simulink model "stdp_pattern3x3_training_2023noclock"  (R2024a)
settings: Solver=FixedStepAuto  StartTime=0.0  StopTime=2  FixedStep=0.000005  RelTol=1e-3
model workspace (MAT data in the model file):
  part1_v1 = 1
values from neighbouring files (symbols this model uses):
  full_pattern = load('Pattern4_250.CSV')    [model_setup4.m]
  max_weight2 = 255    [model_setup4.m]
  min_weight2 = 150    [model_setup4.m]
  Th_control_time2 = 0.02    [model_setup4.m]    (also in model_setup_test.m = 2)
  Th_minus_count2 = 10    [model_setup4.m]    (also in model_setup_test.m = 5)
  Th_plus_count2 = 20    [model_setup4.m]    (also in model_setup_test.m)
libraries: simulink x1
(part 3 of 9)

== system stdp_pattern3x3_training_2023noclock/Synapse22 ==
  note: weight 초기값
  note: pre spike trace
  note: weight 최댓값
  note: STDP
  note: Synapse
  note: weight 최솟값
  note: post spike trace
  note: 기존 weight + STDP 변화량
  note: weight RC 감소
  Pre_spike : Inport
  addr : Inport  Port=2
  Post_spike : Inport  Port=3
  Add1 : Sum
  Clock1 : Subsystem
  Clock2 : Subsystem
  Clock3 : Subsystem
  Delay1 : Delay  DelayLength=1  SampleTime=0.00001
  Exp : Math
  Exp1 : Math
  From Workspace : FromWorkspace  VariableName=Rand_var
  From Workspace1 : FromWorkspace  VariableName=min_weight
  From Workspace2 : FromWorkspace  VariableName=max_weight
  From Workspace3 : FromWorkspace  VariableName=synapse_weight_rc_s
  From Workspace4 : FromWorkspace  VariableName=synapse_weight_rc_l
  From Workspace6 : FromWorkspace  VariableName=initial_LTP
  From Workspace7 : FromWorkspace  VariableName=initial_LTD
  From Workspace8 : FromWorkspace  VariableName=RC_LTP
  From Workspace9 : FromWorkspace  VariableName=RC_LTD
  Gain1 : Gain  Gain=-1
  MATLAB Function1 : MATLAB Function  TreatAsAtomicUnit=on
  Memory1 : Memory
  Memory2 : Memory
  OR : Logic  Operator=OR  IconShape=distinctive  AllPortsSameDT=off  OutDataTypeStr=boolean
  Product{,1..6} (7 alike) : Product
  Scope1 : Scope  NumInputPorts=4
  Scope2 : Scope  NumInputPorts=5
  Scope3 : Scope  NumInputPorts=2
  Scope5 : Scope  NumInputPorts=3
  Scope6 : Scope  NumInputPorts=3
  Scope7 : Scope  NumInputPorts=3
  Scope8 : Scope  NumInputPorts=4
  Subsystem : Subsystem
  Switch : Switch  Threshold=max_weight2  SaturateOnIntegerOverflow=off  InputSameDT=off
  Switch1 : Switch  Criteria=u2 > Threshold  Threshold=min_weight2  SaturateOnIntegerOverflow=off  InputSameDT=off
  rc_add1 : MATLAB Function  TreatAsAtomicUnit=on
  rc_add2 : MATLAB Function  TreatAsAtomicUnit=on
  Weight : Outport
  Spike_out : Outport  Port=2
  Weight_out : Outport  Port=3
  wires:
  Switch1/1 -> Scope7/3, Product/2, Weight_out/1, Scope5/3, Scope3/1, Delay1/1
  Product/1 -> Memory1/1
  addr/1 -> MATLAB Function1/2(synapse_num)
  Post_spike/1 -> Scope2/4, Memory2/1
  Clock1/1(T) -> rc_add2/1(tx)
  Clock2/1(T) -> Scope2/3, rc_add1/1(ty)
  Delay1/1 -> Scope3/2, Subsystem/2(before_weight), Scope6/3
  Memory1/1 -> Weight/1, Scope5/2
  From Workspace7/1 -> rc_add1/2(initial_LTD)
  From Workspace9/1 -> rc_add1/3(tau_LTD)
  From Workspace6/1 -> rc_add2/2(initial_LTP)
  From Workspace8/1 -> rc_add2/3(tau_LTP)
  Product6/1 -> Scope1/4, Add1/2
  Product5/1 -> Scope1/2, Add1/1
  Add1/1 -> Subsystem/1(delta_weight), Scope2/1, Scope6/1
  From Workspace2/1 -> Product3/2
  Product2/1 -> Exp1/1
  Gain1/1 -> Product1/2, Product2/1
  From Workspace1/1 -> Switch1/3
  Exp1/1 -> Scope8/2, Product4/2
  Switch/1 -> Scope8/4, Switch1/2, Scope7/2, Switch1/1
  From Workspace3/1 -> Product2/2
  Product3/1 -> Switch/1
  Exp/1 -> Product3/1
  Clock3/1(T) -> Gain1/1
  Product1/1 -> Exp/1
  MATLAB Function1/1(y) -> Scope6/2, Product4/1, Scope7/1, Switch/2, Scope8/1
  From Workspace4/1 -> Product1/1
  From Workspace/1 -> MATLAB Function1/1(init_weight)
  Product4/1 -> Scope8/3, Switch/3
  Subsystem/1(weight) -> MATLAB Function1/3(before_weight)
  rc_add2/1(pre_trace) -> Product5/1, Scope1/1
  rc_add1/1(post_trace) -> Product6/2, Scope1/3
  OR/1 -> Subsystem/Trigger
  Memory2/1 -> OR/2, Product5/2, Clock2/1("Reset "), Scope2/5
  Pre_spike/1 -> OR/1, Scope5/1, Spike_out/1, Product/1, Clock3/1("Reset "), Clock1/1("Reset "), Product6/1, Scope2/2

== system stdp_pattern3x3_training_2023noclock/Synapse23 ==
  note: weight 초기값
  note: pre spike trace
  note: weight 최댓값
  note: STDP
  note: Synapse
  note: weight 최솟값
  note: post spike trace
  note: 기존 weight + STDP 변화량
  note: weight RC 감소
  Pre_spike : Inport
  addr : Inport  Port=2
  Post_spike : Inport  Port=3
  Add1 : Sum
  Clock1 : Subsystem
  Clock2 : Subsystem
  Clock3 : Subsystem
  Delay1 : Delay  DelayLength=1  SampleTime=0.00001
  Exp : Math
  Exp1 : Math
  From Workspace : FromWorkspace  VariableName=Rand_var
  From Workspace1 : FromWorkspace  VariableName=min_weight
  From Workspace2 : FromWorkspace  VariableName=max_weight
  From Workspace3 : FromWorkspace  VariableName=synapse_weight_rc_s
  From Workspace4 : FromWorkspace  VariableName=synapse_weight_rc_l
  From Workspace6 : FromWorkspace  VariableName=initial_LTP
  From Workspace7 : FromWorkspace  VariableName=initial_LTD
  From Workspace8 : FromWorkspace  VariableName=RC_LTP
  From Workspace9 : FromWorkspace  VariableName=RC_LTD
  Gain1 : Gain  Gain=-1
  MATLAB Function1 : MATLAB Function  TreatAsAtomicUnit=on
  Memory1 : Memory
  Memory2 : Memory
  OR : Logic  Operator=OR  IconShape=distinctive  AllPortsSameDT=off  OutDataTypeStr=boolean
  Product{,1..6} (7 alike) : Product
  Scope1 : Scope  NumInputPorts=4
  Scope2 : Scope  NumInputPorts=5
  Scope3 : Scope  NumInputPorts=2
  Scope5 : Scope  NumInputPorts=3
  Scope6 : Scope  NumInputPorts=3
  Scope7 : Scope  NumInputPorts=3
  Scope8 : Scope  NumInputPorts=4
  Subsystem : Subsystem
  Switch : Switch  Threshold=max_weight2  SaturateOnIntegerOverflow=off  InputSameDT=off
  Switch1 : Switch  Criteria=u2 > Threshold  Threshold=min_weight2  SaturateOnIntegerOverflow=off  InputSameDT=off
  rc_add1 : MATLAB Function  TreatAsAtomicUnit=on
  rc_add2 : MATLAB Function  TreatAsAtomicUnit=on
  Weight : Outport
  Spike_out : Outport  Port=2
  Weight_out : Outport  Port=3
  wires:
  Switch1/1 -> Scope7/3, Product/2, Weight_out/1, Scope5/3, Scope3/1, Delay1/1
  Product/1 -> Memory1/1
  addr/1 -> MATLAB Function1/2(synapse_num)
  Post_spike/1 -> Scope2/4, Memory2/1
  Clock1/1(T) -> rc_add2/1(tx)
  Clock2/1(T) -> Scope2/3, rc_add1/1(ty)
  Delay1/1 -> Scope3/2, Subsystem/2(before_weight), Scope6/3
  Memory1/1 -> Weight/1, Scope5/2
  From Workspace7/1 -> rc_add1/2(initial_LTD)
  From Workspace9/1 -> rc_add1/3(tau_LTD)
  From Workspace6/1 -> rc_add2/2(initial_LTP)
  From Workspace8/1 -> rc_add2/3(tau_LTP)
  Product6/1 -> Scope1/4, Add1/2
  Product5/1 -> Scope1/2, Add1/1
  Add1/1 -> Subsystem/1(delta_weight), Scope2/1, Scope6/1
  From Workspace2/1 -> Product3/2
  Product2/1 -> Exp1/1
  Gain1/1 -> Product1/2, Product2/1
  From Workspace1/1 -> Switch1/3
  Exp1/1 -> Scope8/2, Product4/2
  Switch/1 -> Scope8/4, Switch1/2, Scope7/2, Switch1/1
  From Workspace3/1 -> Product2/2
  Product3/1 -> Switch/1
  Exp/1 -> Product3/1
  Clock3/1(T) -> Gain1/1
  Product1/1 -> Exp/1
  MATLAB Function1/1(y) -> Scope6/2, Product4/1, Scope7/1, Switch/2, Scope8/1
  From Workspace4/1 -> Product1/1
  From Workspace/1 -> MATLAB Function1/1(init_weight)
  Product4/1 -> Scope8/3, Switch/3
  Subsystem/1(weight) -> MATLAB Function1/3(before_weight)
  rc_add2/1(pre_trace) -> Product5/1, Scope1/1
  rc_add1/1(post_trace) -> Product6/2, Scope1/3
  OR/1 -> Subsystem/Trigger
  Memory2/1 -> OR/2, Product5/2, Clock2/1("Reset "), Scope2/5
  Pre_spike/1 -> OR/1, Scope5/1, Spike_out/1, Product/1, Clock3/1("Reset "), Clock1/1("Reset "), Product6/1, Scope2/2

== system stdp_pattern3x3_training_2023noclock/Synapse24 ==
  note: weight 초기값
  note: pre spike trace
  note: weight 최댓값
  note: STDP
  note: Synapse
  note: weight 최솟값
  note: post spike trace
  note: 기존 weight + STDP 변화량
  note: weight RC 감소
  Pre_spike : Inport
  addr : Inport  Port=2
  Post_spike : Inport  Port=3
  Add1 : Sum
  Clock1 : Subsystem
  Clock2 : Subsystem
  Clock3 : Subsystem
  Delay1 : Delay  DelayLength=1  SampleTime=0.00001
  Exp : Math
  Exp1 : Math
  From Workspace : FromWorkspace  VariableName=Rand_var
  From Workspace1 : FromWorkspace  VariableName=min_weight
  From Workspace2 : FromWorkspace  VariableName=max_weight
  From Workspace3 : FromWorkspace  VariableName=synapse_weight_rc_s
  From Workspace4 : FromWorkspace  VariableName=synapse_weight_rc_l
  From Workspace6 : FromWorkspace  VariableName=initial_LTP
  From Workspace7 : FromWorkspace  VariableName=initial_LTD
  From Workspace8 : FromWorkspace  VariableName=RC_LTP
  From Workspace9 : FromWorkspace  VariableName=RC_LTD
  Gain1 : Gain  Gain=-1
  MATLAB Function1 : MATLAB Function  TreatAsAtomicUnit=on
  Memory1 : Memory
  Memory2 : Memory
  OR : Logic  Operator=OR  IconShape=distinctive  AllPortsSameDT=off  OutDataTypeStr=boolean
  Product{,1..6} (7 alike) : Product
  Scope1 : Scope  NumInputPorts=4
  Scope2 : Scope  NumInputPorts=5
  Scope3 : Scope  NumInputPorts=2
  Scope5 : Scope  NumInputPorts=3
  Scope6 : Scope  NumInputPorts=3
  Scope7 : Scope  NumInputPorts=3
  Scope8 : Scope  NumInputPorts=4
  Subsystem : Subsystem
  Switch : Switch  Threshold=max_weight2  SaturateOnIntegerOverflow=off  InputSameDT=off
  Switch1 : Switch  Criteria=u2 > Threshold  Threshold=min_weight2  SaturateOnIntegerOverflow=off  InputSameDT=off
  rc_add1 : MATLAB Function  TreatAsAtomicUnit=on
  rc_add2 : MATLAB Function  TreatAsAtomicUnit=on
  Weight : Outport
  Spike_out : Outport  Port=2
  Weight_out : Outport  Port=3
  wires:
  Switch1/1 -> Scope7/3, Product/2, Weight_out/1, Scope5/3, Scope3/1, Delay1/1
  Product/1 -> Memory1/1
  addr/1 -> MATLAB Function1/2(synapse_num)
  Post_spike/1 -> Scope2/4, Memory2/1
  Clock1/1(T) -> rc_add2/1(tx)
  Clock2/1(T) -> Scope2/3, rc_add1/1(ty)
  Delay1/1 -> Scope3/2, Subsystem/2(before_weight), Scope6/3
  Memory1/1 -> Weight/1, Scope5/2
  From Workspace7/1 -> rc_add1/2(initial_LTD)
  From Workspace9/1 -> rc_add1/3(tau_LTD)
  From Workspace6/1 -> rc_add2/2(initial_LTP)
  From Workspace8/1 -> rc_add2/3(tau_LTP)
  Product6/1 -> Scope1/4, Add1/2
  Product5/1 -> Scope1/2, Add1/1
  Add1/1 -> Subsystem/1(delta_weight), Scope2/1, Scope6/1
  From Workspace2/1 -> Product3/2
  Product2/1 -> Exp1/1
  Gain1/1 -> Product1/2, Product2/1
  From Workspace1/1 -> Switch1/3
  Exp1/1 -> Scope8/2, Product4/2
  Switch/1 -> Scope8/4, Switch1/2, Scope7/2, Switch1/1
  From Workspace3/1 -> Product2/2
  Product3/1 -> Switch/1
  Exp/1 -> Product3/1
  Clock3/1(T) -> Gain1/1
  Product1/1 -> Exp/1
  MATLAB Function1/1(y) -> Scope6/2, Product4/1, Scope7/1, Switch/2, Scope8/1
  From Workspace4/1 -> Product1/1
  From Workspace/1 -> MATLAB Function1/1(init_weight)
  Product4/1 -> Scope8/3, Switch/3
  Subsystem/1(weight) -> MATLAB Function1/3(before_weight)
  rc_add2/1(pre_trace) -> Product5/1, Scope1/1
  rc_add1/1(post_trace) -> Product6/2, Scope1/3
  OR/1 -> Subsystem/Trigger
  Memory2/1 -> OR/2, Product5/2, Clock2/1("Reset "), Scope2/5
  Pre_spike/1 -> OR/1, Scope5/1, Spike_out/1, Product/1, Clock3/1("Reset "), Clock1/1("Reset "), Product6/1, Scope2/2

== system stdp_pattern3x3_training_2023noclock/Synapse25 ==
  note: weight 초기값
  note: pre spike trace
  note: weight 최댓값
  note: STDP
  note: Synapse
  note: weight 최솟값
  note: post spike trace
  note: 기존 weight + STDP 변화량
  note: weight RC 감소
  Pre_spike : Inport
  addr : Inport  Port=2
  Post_spike : Inport  Port=3
  Add1 : Sum
  Clock1 : Subsystem
  Clock2 : Subsystem
  Clock3 : Subsystem
  Delay1 : Delay  DelayLength=1  SampleTime=0.00001
  Exp : Math
  Exp1 : Math
  From Workspace : FromWorkspace  VariableName=Rand_var
  From Workspace1 : FromWorkspace  VariableName=min_weight
  From Workspace2 : FromWorkspace  VariableName=max_weight
  From Workspace3 : FromWorkspace  VariableName=synapse_weight_rc_s
  From Workspace4 : FromWorkspace  VariableName=synapse_weight_rc_l
  From Workspace6 : FromWorkspace  VariableName=initial_LTP
  From Workspace7 : FromWorkspace  VariableName=initial_LTD
  From Workspace8 : FromWorkspace  VariableName=RC_LTP
  From Workspace9 : FromWorkspace  VariableName=RC_LTD
  Gain1 : Gain  Gain=-1
  MATLAB Function1 : MATLAB Function  TreatAsAtomicUnit=on
  Memory1 : Memory
  Memory2 : Memory
  OR : Logic  Operator=OR  IconShape=distinctive  AllPortsSameDT=off  OutDataTypeStr=boolean
  Product{,1..6} (7 alike) : Product
  Scope1 : Scope  NumInputPorts=4
  Scope2 : Scope  NumInputPorts=5
  Scope3 : Scope  NumInputPorts=2
  Scope5 : Scope  NumInputPorts=3
  Scope6 : Scope  NumInputPorts=3
  Scope7 : Scope  NumInputPorts=3
  Scope8 : Scope  NumInputPorts=4
  Subsystem : Subsystem
  Switch : Switch  Threshold=max_weight2  SaturateOnIntegerOverflow=off  InputSameDT=off
  Switch1 : Switch  Criteria=u2 > Threshold  Threshold=min_weight2  SaturateOnIntegerOverflow=off  InputSameDT=off
  rc_add1 : MATLAB Function  TreatAsAtomicUnit=on
  rc_add2 : MATLAB Function  TreatAsAtomicUnit=on
  Weight : Outport
  Spike_out : Outport  Port=2
  Weight_out : Outport  Port=3
  wires:
  Switch1/1 -> Scope7/3, Product/2, Weight_out/1, Scope5/3, Scope3/1, Delay1/1
  Product/1 -> Memory1/1
  addr/1 -> MATLAB Function1/2(synapse_num)
  Post_spike/1 -> Scope2/4, Memory2/1
  Clock1/1(T) -> rc_add2/1(tx)
  Clock2/1(T) -> Scope2/3, rc_add1/1(ty)
  Delay1/1 -> Scope3/2, Subsystem/2(before_weight), Scope6/3
  Memory1/1 -> Weight/1, Scope5/2
  From Workspace7/1 -> rc_add1/2(initial_LTD)
  From Workspace9/1 -> rc_add1/3(tau_LTD)
  From Workspace6/1 -> rc_add2/2(initial_LTP)
  From Workspace8/1 -> rc_add2/3(tau_LTP)
  Product6/1 -> Scope1/4, Add1/2
  Product5/1 -> Scope1/2, Add1/1
  Add1/1 -> Subsystem/1(delta_weight), Scope2/1, Scope6/1
  From Workspace2/1 -> Product3/2
  Product2/1 -> Exp1/1
  Gain1/1 -> Product1/2, Product2/1
  From Workspace1/1 -> Switch1/3
  Exp1/1 -> Scope8/2, Product4/2
  Switch/1 -> Scope8/4, Switch1/2, Scope7/2, Switch1/1
  From Workspace3/1 -> Product2/2
  Product3/1 -> Switch/1
  Exp/1 -> Product3/1
  Clock3/1(T) -> Gain1/1
  Product1/1 -> Exp/1
  MATLAB Function1/1(y) -> Scope6/2, Product4/1, Scope7/1, Switch/2, Scope8/1
  From Workspace4/1 -> Product1/1
  From Workspace/1 -> MATLAB Function1/1(init_weight)
  Product4/1 -> Scope8/3, Switch/3
  Subsystem/1(weight) -> MATLAB Function1/3(before_weight)
  rc_add2/1(pre_trace) -> Product5/1, Scope1/1
  rc_add1/1(post_trace) -> Product6/2, Scope1/3
  OR/1 -> Subsystem/Trigger
  Memory2/1 -> OR/2, Product5/2, Clock2/1("Reset "), Scope2/5
  Pre_spike/1 -> OR/1, Scope5/1, Spike_out/1, Product/1, Clock3/1("Reset "), Clock1/1("Reset "), Product6/1, Scope2/2

== system stdp_pattern3x3_training_2023noclock/Synapse26 ==
  note: weight 초기값
  note: pre spike trace
  note: weight 최댓값
  note: STDP
  note: Synapse
  note: weight 최솟값
  note: post spike trace
  note: 기존 weight + STDP 변화량
  note: weight RC 감소
  Pre_spike : Inport
  addr : Inport  Port=2
  Post_spike : Inport  Port=3
  Add1 : Sum
  Clock1 : Subsystem
  Clock2 : Subsystem
  Clock3 : Subsystem
  Delay1 : Delay  DelayLength=1  SampleTime=0.00001
  Exp : Math
  Exp1 : Math
  From Workspace : FromWorkspace  VariableName=Rand_var
  From Workspace1 : FromWorkspace  VariableName=min_weight
  From Workspace2 : FromWorkspace  VariableName=max_weight
  From Workspace3 : FromWorkspace  VariableName=synapse_weight_rc_s
  From Workspace4 : FromWorkspace  VariableName=synapse_weight_rc_l
  From Workspace6 : FromWorkspace  VariableName=initial_LTP
  From Workspace7 : FromWorkspace  VariableName=initial_LTD
  From Workspace8 : FromWorkspace  VariableName=RC_LTP
  From Workspace9 : FromWorkspace  VariableName=RC_LTD
  Gain1 : Gain  Gain=-1
  MATLAB Function1 : MATLAB Function  TreatAsAtomicUnit=on
  Memory1 : Memory
  Memory2 : Memory
  OR : Logic  Operator=OR  IconShape=distinctive  AllPortsSameDT=off  OutDataTypeStr=boolean
  Product{,1..6} (7 alike) : Product
  Scope1 : Scope  NumInputPorts=4
  Scope2 : Scope  NumInputPorts=5
  Scope3 : Scope  NumInputPorts=2
  Scope5 : Scope  NumInputPorts=3
  Scope6 : Scope  NumInputPorts=3
  Scope7 : Scope  NumInputPorts=3
  Scope8 : Scope  NumInputPorts=4
  Subsystem : Subsystem
  Switch : Switch  Threshold=max_weight2  SaturateOnIntegerOverflow=off  InputSameDT=off
  Switch1 : Switch  Criteria=u2 > Threshold  Threshold=min_weight2  SaturateOnIntegerOverflow=off  InputSameDT=off
  rc_add1 : MATLAB Function  TreatAsAtomicUnit=on
  rc_add2 : MATLAB Function  TreatAsAtomicUnit=on
  Weight : Outport
  Spike_out : Outport  Port=2
  Weight_out : Outport  Port=3
  wires:
  Switch1/1 -> Scope7/3, Product/2, Weight_out/1, Scope5/3, Scope3/1, Delay1/1
  Product/1 -> Memory1/1
  addr/1 -> MATLAB Function1/2(synapse_num)
  Post_spike/1 -> Scope2/4, Memory2/1
  Clock1/1(T) -> rc_add2/1(tx)
  Clock2/1(T) -> Scope2/3, rc_add1/1(ty)
  Delay1/1 -> Scope3/2, Subsystem/2(before_weight), Scope6/3
  Memory1/1 -> Weight/1, Scope5/2
  From Workspace7/1 -> rc_add1/2(initial_LTD)
  From Workspace9/1 -> rc_add1/3(tau_LTD)
  From Workspace6/1 -> rc_add2/2(initial_LTP)
  From Workspace8/1 -> rc_add2/3(tau_LTP)
  Product6/1 -> Scope1/4, Add1/2
  Product5/1 -> Scope1/2, Add1/1
  Add1/1 -> Subsystem/1(delta_weight), Scope2/1, Scope6/1
  From Workspace2/1 -> Product3/2
  Product2/1 -> Exp1/1
  Gain1/1 -> Product1/2, Product2/1
  From Workspace1/1 -> Switch1/3
  Exp1/1 -> Scope8/2, Product4/2
  Switch/1 -> Scope8/4, Switch1/2, Scope7/2, Switch1/1
  From Workspace3/1 -> Product2/2
  Product3/1 -> Switch/1
  Exp/1 -> Product3/1
  Clock3/1(T) -> Gain1/1
  Product1/1 -> Exp/1
  MATLAB Function1/1(y) -> Scope6/2, Product4/1, Scope7/1, Switch/2, Scope8/1
  From Workspace4/1 -> Product1/1
  From Workspace/1 -> MATLAB Function1/1(init_weight)
  Product4/1 -> Scope8/3, Switch/3
  Subsystem/1(weight) -> MATLAB Function1/3(before_weight)
  rc_add2/1(pre_trace) -> Product5/1, Scope1/1
  rc_add1/1(post_trace) -> Product6/2, Scope1/3
  OR/1 -> Subsystem/Trigger
  Memory2/1 -> OR/2, Product5/2, Clock2/1("Reset "), Scope2/5
  Pre_spike/1 -> OR/1, Scope5/1, Spike_out/1, Product/1, Clock3/1("Reset "), Clock1/1("Reset "), Product6/1, Scope2/2

== system stdp_pattern3x3_training_2023noclock/Synapse27 ==
  note: weight 초기값
  note: pre spike trace
  note: weight 최댓값
  note: STDP
  note: Synapse
  note: weight 최솟값
  note: post spike trace
  note: 기존 weight + STDP 변화량
  note: weight RC 감소
  Pre_spike : Inport
  addr : Inport  Port=2
  Post_spike : Inport  Port=3
  Add1 : Sum
  Clock1 : Subsystem
  Clock2 : Subsystem
  Clock3 : Subsystem
  Delay1 : Delay  DelayLength=1  SampleTime=0.00001
  Exp : Math
  Exp1 : Math
  From Workspace : FromWorkspace  VariableName=Rand_var
  From Workspace1 : FromWorkspace  VariableName=min_weight
  From Workspace2 : FromWorkspace  VariableName=max_weight
  From Workspace3 : FromWorkspace  VariableName=synapse_weight_rc_s
  From Workspace4 : FromWorkspace  VariableName=synapse_weight_rc_l
  From Workspace6 : FromWorkspace  VariableName=initial_LTP
  From Workspace7 : FromWorkspace  VariableName=initial_LTD
  From Workspace8 : FromWorkspace  VariableName=RC_LTP
  From Workspace9 : FromWorkspace  VariableName=RC_LTD
  Gain1 : Gain  Gain=-1
  MATLAB Function1 : MATLAB Function  TreatAsAtomicUnit=on
  Memory1 : Memory
  Memory2 : Memory
  OR : Logic  Operator=OR  IconShape=distinctive  AllPortsSameDT=off  OutDataTypeStr=boolean
  Product{,1..6} (7 alike) : Product
  Scope1 : Scope  NumInputPorts=4
  Scope2 : Scope  NumInputPorts=5
  Scope3 : Scope  NumInputPorts=2
  Scope5 : Scope  NumInputPorts=3
  Scope6 : Scope  NumInputPorts=3
  Scope7 : Scope  NumInputPorts=3
  Scope8 : Scope  NumInputPorts=4
  Subsystem : Subsystem
  Switch : Switch  Threshold=max_weight2  SaturateOnIntegerOverflow=off  InputSameDT=off
  Switch1 : Switch  Criteria=u2 > Threshold  Threshold=min_weight2  SaturateOnIntegerOverflow=off  InputSameDT=off
  rc_add1 : MATLAB Function  TreatAsAtomicUnit=on
  rc_add2 : MATLAB Function  TreatAsAtomicUnit=on
  Weight : Outport
  Spike_out : Outport  Port=2
  Weight_out : Outport  Port=3
  wires:
  Switch1/1 -> Scope7/3, Product/2, Weight_out/1, Scope5/3, Scope3/1, Delay1/1
  Product/1 -> Memory1/1
  addr/1 -> MATLAB Function1/2(synapse_num)
  Post_spike/1 -> Scope2/4, Memory2/1
  Clock1/1(T) -> rc_add2/1(tx)
  Clock2/1(T) -> Scope2/3, rc_add1/1(ty)
  Delay1/1 -> Scope3/2, Subsystem/2(before_weight), Scope6/3
  Memory1/1 -> Weight/1, Scope5/2
  From Workspace7/1 -> rc_add1/2(initial_LTD)
  From Workspace9/1 -> rc_add1/3(tau_LTD)
  From Workspace6/1 -> rc_add2/2(initial_LTP)
  From Workspace8/1 -> rc_add2/3(tau_LTP)
  Product6/1 -> Scope1/4, Add1/2
  Product5/1 -> Scope1/2, Add1/1
  Add1/1 -> Subsystem/1(delta_weight), Scope2/1, Scope6/1
  From Workspace2/1 -> Product3/2
  Product2/1 -> Exp1/1
  Gain1/1 -> Product1/2, Product2/1
  From Workspace1/1 -> Switch1/3
  Exp1/1 -> Scope8/2, Product4/2
  Switch/1 -> Scope8/4, Switch1/2, Scope7/2, Switch1/1
  From Workspace3/1 -> Product2/2
  Product3/1 -> Switch/1
  Exp/1 -> Product3/1
  Clock3/1(T) -> Gain1/1
  Product1/1 -> Exp/1
  MATLAB Function1/1(y) -> Scope6/2, Product4/1, Scope7/1, Switch/2, Scope8/1
  From Workspace4/1 -> Product1/1
  From Workspace/1 -> MATLAB Function1/1(init_weight)
  Product4/1 -> Scope8/3, Switch/3
  Subsystem/1(weight) -> MATLAB Function1/3(before_weight)
  rc_add2/1(pre_trace) -> Product5/1, Scope1/1
  rc_add1/1(post_trace) -> Product6/2, Scope1/3
  OR/1 -> Subsystem/Trigger
  Memory2/1 -> OR/2, Product5/2, Clock2/1("Reset "), Scope2/5
  Pre_spike/1 -> OR/1, Scope5/1, Spike_out/1, Product/1, Clock3/1("Reset "), Clock1/1("Reset "), Product6/1, Scope2/2

== system stdp_pattern3x3_training_2023noclock/Synapse28 ==
  note: weight 초기값
  note: pre spike trace
  note: weight 최댓값
  note: STDP
  note: Synapse
  note: weight 최솟값
  note: post spike trace
  note: 기존 weight + STDP 변화량
  note: weight RC 감소
  Pre_spike : Inport
  addr : Inport  Port=2
  Post_spike : Inport  Port=3
  Add1 : Sum
  Clock1 : Subsystem
  Clock2 : Subsystem
  Clock3 : Subsystem
  Delay1 : Delay  DelayLength=1  SampleTime=0.00001
  Exp : Math
  Exp1 : Math
  From Workspace : FromWorkspace  VariableName=Rand_var
  From Workspace1 : FromWorkspace  VariableName=min_weight
  From Workspace2 : FromWorkspace  VariableName=max_weight
  From Workspace3 : FromWorkspace  VariableName=synapse_weight_rc_s
  From Workspace4 : FromWorkspace  VariableName=synapse_weight_rc_l
  From Workspace6 : FromWorkspace  VariableName=initial_LTP
  From Workspace7 : FromWorkspace  VariableName=initial_LTD
  From Workspace8 : FromWorkspace  VariableName=RC_LTP
  From Workspace9 : FromWorkspace  VariableName=RC_LTD
  Gain1 : Gain  Gain=-1
  MATLAB Function1 : MATLAB Function  TreatAsAtomicUnit=on
  Memory1 : Memory
  Memory2 : Memory
  OR : Logic  Operator=OR  IconShape=distinctive  AllPortsSameDT=off  OutDataTypeStr=boolean
  Product{,1..6} (7 alike) : Product
  Scope1 : Scope  NumInputPorts=4
  Scope2 : Scope  NumInputPorts=5
  Scope3 : Scope  NumInputPorts=2
  Scope5 : Scope  NumInputPorts=3
  Scope6 : Scope  NumInputPorts=3
  Scope7 : Scope  NumInputPorts=3
  Scope8 : Scope  NumInputPorts=4
  Subsystem : Subsystem
  Switch : Switch  Threshold=max_weight2  SaturateOnIntegerOverflow=off  InputSameDT=off
  Switch1 : Switch  Criteria=u2 > Threshold  Threshold=min_weight2  SaturateOnIntegerOverflow=off  InputSameDT=off
  rc_add1 : MATLAB Function  TreatAsAtomicUnit=on
  rc_add2 : MATLAB Function  TreatAsAtomicUnit=on
  Weight : Outport
  Spike_out : Outport  Port=2
  Weight_out : Outport  Port=3
  wires:
  Switch1/1 -> Scope7/3, Product/2, Weight_out/1, Scope5/3, Scope3/1, Delay1/1
  Product/1 -> Memory1/1
  addr/1 -> MATLAB Function1/2(synapse_num)
  Post_spike/1 -> Scope2/4, Memory2/1
  Clock1/1(T) -> rc_add2/1(tx)
  Clock2/1(T) -> Scope2/3, rc_add1/1(ty)
  Delay1/1 -> Scope3/2, Subsystem/2(before_weight), Scope6/3
  Memory1/1 -> Weight/1, Scope5/2
  From Workspace7/1 -> rc_add1/2(initial_LTD)
  From Workspace9/1 -> rc_add1/3(tau_LTD)
  From Workspace6/1 -> rc_add2/2(initial_LTP)
  From Workspace8/1 -> rc_add2/3(tau_LTP)
  Product6/1 -> Scope1/4, Add1/2
  Product5/1 -> Scope1/2, Add1/1
  Add1/1 -> Subsystem/1(delta_weight), Scope2/1, Scope6/1
  From Workspace2/1 -> Product3/2
  Product2/1 -> Exp1/1
  Gain1/1 -> Product1/2, Product2/1
  From Workspace1/1 -> Switch1/3
  Exp1/1 -> Scope8/2, Product4/2
  Switch/1 -> Scope8/4, Switch1/2, Scope7/2, Switch1/1
  From Workspace3/1 -> Product2/2
  Product3/1 -> Switch/1
  Exp/1 -> Product3/1
  Clock3/1(T) -> Gain1/1
  Product1/1 -> Exp/1
  MATLAB Function1/1(y) -> Scope6/2, Product4/1, Scope7/1, Switch/2, Scope8/1
  From Workspace4/1 -> Product1/1
  From Workspace/1 -> MATLAB Function1/1(init_weight)
  Product4/1 -> Scope8/3, Switch/3
  Subsystem/1(weight) -> MATLAB Function1/3(before_weight)
  rc_add2/1(pre_trace) -> Product5/1, Scope1/1
  rc_add1/1(post_trace) -> Product6/2, Scope1/3
  OR/1 -> Subsystem/Trigger
  Memory2/1 -> OR/2, Product5/2, Clock2/1("Reset "), Scope2/5
  Pre_spike/1 -> OR/1, Scope5/1, Spike_out/1, Product/1, Clock3/1("Reset "), Clock1/1("Reset "), Product6/1, Scope2/2

== system stdp_pattern3x3_training_2023noclock/Synapse29 ==
  note: weight 초기값
  note: pre spike trace
  note: weight 최댓값
  note: STDP
  note: Synapse
  note: weight 최솟값
  note: post spike trace
  note: 기존 weight + STDP 변화량
  note: weight RC 감소
  Pre_spike : Inport
  addr : Inport  Port=2
  Post_spike : Inport  Port=3
  Add1 : Sum
  Clock1 : Subsystem
  Clock2 : Subsystem
  Clock3 : Subsystem
  Delay1 : Delay  DelayLength=1  SampleTime=0.00001
  Exp : Math
  Exp1 : Math
  From Workspace : FromWorkspace  VariableName=Rand_var
  From Workspace1 : FromWorkspace  VariableName=min_weight
  From Workspace2 : FromWorkspace  VariableName=max_weight
  From Workspace3 : FromWorkspace  VariableName=synapse_weight_rc_s
  From Workspace4 : FromWorkspace  VariableName=synapse_weight_rc_l
  From Workspace6 : FromWorkspace  VariableName=initial_LTP
  From Workspace7 : FromWorkspace  VariableName=initial_LTD
  From Workspace8 : FromWorkspace  VariableName=RC_LTP
  From Workspace9 : FromWorkspace  VariableName=RC_LTD
  Gain1 : Gain  Gain=-1
  MATLAB Function1 : MATLAB Function  TreatAsAtomicUnit=on
  Memory1 : Memory
  Memory2 : Memory
  OR : Logic  Operator=OR  IconShape=distinctive  AllPortsSameDT=off  OutDataTypeStr=boolean
  Product{,1..6} (7 alike) : Product
  Scope1 : Scope  NumInputPorts=4
  Scope2 : Scope  NumInputPorts=5
  Scope3 : Scope  NumInputPorts=2
  Scope5 : Scope  NumInputPorts=3
  Scope6 : Scope  NumInputPorts=3
  Scope7 : Scope  NumInputPorts=3
  Scope8 : Scope  NumInputPorts=4
  Subsystem : Subsystem
  Switch : Switch  Threshold=max_weight2  SaturateOnIntegerOverflow=off  InputSameDT=off
  Switch1 : Switch  Criteria=u2 > Threshold  Threshold=min_weight2  SaturateOnIntegerOverflow=off  InputSameDT=off
  rc_add1 : MATLAB Function  TreatAsAtomicUnit=on
  rc_add2 : MATLAB Function  TreatAsAtomicUnit=on
  Weight : Outport
  Spike_out : Outport  Port=2
  Weight_out : Outport  Port=3
  wires:
  Switch1/1 -> Scope7/3, Product/2, Weight_out/1, Scope5/3, Scope3/1, Delay1/1
  Product/1 -> Memory1/1
  addr/1 -> MATLAB Function1/2(synapse_num)
  Post_spike/1 -> Scope2/4, Memory2/1
  Clock1/1(T) -> rc_add2/1(tx)
  Clock2/1(T) -> Scope2/3, rc_add1/1(ty)
  Delay1/1 -> Scope3/2, Subsystem/2(before_weight), Scope6/3
  Memory1/1 -> Weight/1, Scope5/2
  From Workspace7/1 -> rc_add1/2(initial_LTD)
  From Workspace9/1 -> rc_add1/3(tau_LTD)
  From Workspace6/1 -> rc_add2/2(initial_LTP)
  From Workspace8/1 -> rc_add2/3(tau_LTP)
  Product6/1 -> Scope1/4, Add1/2
  Product5/1 -> Scope1/2, Add1/1
  Add1/1 -> Subsystem/1(delta_weight), Scope2/1, Scope6/1
  From Workspace2/1 -> Product3/2
  Product2/1 -> Exp1/1
  Gain1/1 -> Product1/2, Product2/1
  From Workspace1/1 -> Switch1/3
  Exp1/1 -> Scope8/2, Product4/2
  Switch/1 -> Scope8/4, Switch1/2, Scope7/2, Switch1/1
  From Workspace3/1 -> Product2/2
  Product3/1 -> Switch/1
  Exp/1 -> Product3/1
  Clock3/1(T) -> Gain1/1
  Product1/1 -> Exp/1
  MATLAB Function1/1(y) -> Scope6/2, Product4/1, Scope7/1, Switch/2, Scope8/1
  From Workspace4/1 -> Product1/1
  From Workspace/1 -> MATLAB Function1/1(init_weight)
  Product4/1 -> Scope8/3, Switch/3
  Subsystem/1(weight) -> MATLAB Function1/3(before_weight)
  rc_add2/1(pre_trace) -> Product5/1, Scope1/1
  rc_add1/1(post_trace) -> Product6/2, Scope1/3
  OR/1 -> Subsystem/Trigger
  Memory2/1 -> OR/2, Product5/2, Clock2/1("Reset "), Scope2/5
  Pre_spike/1 -> OR/1, Scope5/1, Spike_out/1, Product/1, Clock3/1("Reset "), Clock1/1("Reset "), Product6/1, Scope2/2

== system stdp_pattern3x3_training_2023noclock/Synapse3 ==
  note: weight 초기값
  note: pre spike trace
  note: weight 최댓값
  note: STDP
  note: Synapse
  note: weight 최솟값
  note: post spike trace
  note: 기존 weight + STDP 변화량
  note: weight RC 감소
  Pre_spike : Inport
  addr : Inport  Port=2
  Post_spike : Inport  Port=3
  Add1 : Sum
  Clock1 : Subsystem
  Clock2 : Subsystem
  Clock3 : Subsystem
  Delay1 : Delay  DelayLength=1  SampleTime=0.00001
  Exp : Math
  Exp1 : Math
  From Workspace : FromWorkspace  VariableName=Rand_var
  From Workspace1 : FromWorkspace  VariableName=min_weight
  From Workspace2 : FromWorkspace  VariableName=max_weight
  From Workspace3 : FromWorkspace  VariableName=synapse_weight_rc_s
  From Workspace4 : FromWorkspace  VariableName=synapse_weight_rc_l
  From Workspace6 : FromWorkspace  VariableName=initial_LTP
  From Workspace7 : FromWorkspace  VariableName=initial_LTD
  From Workspace8 : FromWorkspace  VariableName=RC_LTP
  From Workspace9 : FromWorkspace  VariableName=RC_LTD
  Gain1 : Gain  Gain=-1
  MATLAB Function1 : MATLAB Function  TreatAsAtomicUnit=on
  Memory1 : Memory
  Memory2 : Memory
  OR : Logic  Operator=OR  IconShape=distinctive  AllPortsSameDT=off  OutDataTypeStr=boolean
  Product{,1..6} (7 alike) : Product
  Scope1 : Scope  NumInputPorts=4
  Scope2 : Scope  NumInputPorts=5
  Scope3 : Scope  NumInputPorts=2
  Scope5 : Scope  NumInputPorts=3
  Scope6 : Scope  NumInputPorts=3
  Scope7 : Scope  NumInputPorts=3
  Scope8 : Scope  NumInputPorts=4
  Subsystem : Subsystem
  Switch : Switch  Threshold=max_weight2  SaturateOnIntegerOverflow=off  InputSameDT=off
  Switch1 : Switch  Criteria=u2 > Threshold  Threshold=min_weight2  SaturateOnIntegerOverflow=off  InputSameDT=off
  rc_add1 : MATLAB Function  TreatAsAtomicUnit=on
  rc_add2 : MATLAB Function  TreatAsAtomicUnit=on
  Weight : Outport
  Spike_out : Outport  Port=2
  Weight_out : Outport  Port=3
  wires:
  Switch1/1 -> Scope7/3, Product/2, Weight_out/1, Scope5/3, Scope3/1, Delay1/1
  Product/1 -> Memory1/1
  addr/1 -> MATLAB Function1/2(synapse_num)
  Post_spike/1 -> Scope2/4, Memory2/1
  Clock1/1(T) -> rc_add2/1(tx)
  Clock2/1(T) -> Scope2/3, rc_add1/1(ty)
  Delay1/1 -> Scope3/2, Subsystem/2(before_weight), Scope6/3
  Memory1/1 -> Weight/1, Scope5/2
  From Workspace7/1 -> rc_add1/2(initial_LTD)
  From Workspace9/1 -> rc_add1/3(tau_LTD)
  From Workspace6/1 -> rc_add2/2(initial_LTP)
  From Workspace8/1 -> rc_add2/3(tau_LTP)
  Product6/1 -> Scope1/4, Add1/2
  Product5/1 -> Scope1/2, Add1/1
  Add1/1 -> Subsystem/1(delta_weight), Scope2/1, Scope6/1
  From Workspace2/1 -> Product3/2
  Product2/1 -> Exp1/1
  Gain1/1 -> Product1/2, Product2/1
  From Workspace1/1 -> Switch1/3
  Exp1/1 -> Scope8/2, Product4/2
  Switch/1 -> Scope8/4, Switch1/2, Scope7/2, Switch1/1
  From Workspace3/1 -> Product2/2
  Product3/1 -> Switch/1
  Exp/1 -> Product3/1
  Clock3/1(T) -> Gain1/1
  Product1/1 -> Exp/1
  MATLAB Function1/1(y) -> Scope6/2, Product4/1, Scope7/1, Switch/2, Scope8/1
  From Workspace4/1 -> Product1/1
  From Workspace/1 -> MATLAB Function1/1(init_weight)
  Product4/1 -> Scope8/3, Switch/3
  Subsystem/1(weight) -> MATLAB Function1/3(before_weight)
  rc_add2/1(pre_trace) -> Product5/1, Scope1/1
  rc_add1/1(post_trace) -> Product6/2, Scope1/3
  OR/1 -> Subsystem/Trigger
  Memory2/1 -> OR/2, Product5/2, Clock2/1("Reset "), Scope2/5
  Pre_spike/1 -> OR/1, Scope5/1, Spike_out/1, Product/1, Clock3/1("Reset "), Clock1/1("Reset "), Product6/1, Scope2/2

== system stdp_pattern3x3_training_2023noclock/Synapse30 ==
  note: weight 초기값
  note: pre spike trace
  note: weight 최댓값
  note: STDP
  note: Synapse
  note: weight 최솟값
  note: post spike trace
  note: 기존 weight + STDP 변화량
  note: weight RC 감소
  Pre_spike : Inport
  addr : Inport  Port=2
  Post_spike : Inport  Port=3
  Add1 : Sum
  Clock1 : Subsystem
  Clock2 : Subsystem
  Clock3 : Subsystem
  Delay1 : Delay  DelayLength=1  SampleTime=0.00001
  Exp : Math
  Exp1 : Math
  From Workspace : FromWorkspace  VariableName=Rand_var
  From Workspace1 : FromWorkspace  VariableName=min_weight
  From Workspace2 : FromWorkspace  VariableName=max_weight
  From Workspace3 : FromWorkspace  VariableName=synapse_weight_rc_s
  From Workspace4 : FromWorkspace  VariableName=synapse_weight_rc_l
  From Workspace6 : FromWorkspace  VariableName=initial_LTP
  From Workspace7 : FromWorkspace  VariableName=initial_LTD
  From Workspace8 : FromWorkspace  VariableName=RC_LTP
  From Workspace9 : FromWorkspace  VariableName=RC_LTD
  Gain1 : Gain  Gain=-1
  MATLAB Function1 : MATLAB Function  TreatAsAtomicUnit=on
  Memory1 : Memory
  Memory2 : Memory
  OR : Logic  Operator=OR  IconShape=distinctive  AllPortsSameDT=off  OutDataTypeStr=boolean
  Product{,1..6} (7 alike) : Product
  Scope1 : Scope  NumInputPorts=4
  Scope2 : Scope  NumInputPorts=5
  Scope3 : Scope  NumInputPorts=2
  Scope5 : Scope  NumInputPorts=3
  Scope6 : Scope  NumInputPorts=3
  Scope7 : Scope  NumInputPorts=3
  Scope8 : Scope  NumInputPorts=4
  Subsystem : Subsystem
  Switch : Switch  Threshold=max_weight2  SaturateOnIntegerOverflow=off  InputSameDT=off
  Switch1 : Switch  Criteria=u2 > Threshold  Threshold=min_weight2  SaturateOnIntegerOverflow=off  InputSameDT=off
  rc_add1 : MATLAB Function  TreatAsAtomicUnit=on
  rc_add2 : MATLAB Function  TreatAsAtomicUnit=on
  Weight : Outport
  Spike_out : Outport  Port=2
  Weight_out : Outport  Port=3
  wires:
  Switch1/1 -> Scope7/3, Product/2, Weight_out/1, Scope5/3, Scope3/1, Delay1/1
  Product/1 -> Memory1/1
  addr/1 -> MATLAB Function1/2(synapse_num)
  Post_spike/1 -> Scope2/4, Memory2/1
  Clock1/1(T) -> rc_add2/1(tx)
  Clock2/1(T) -> Scope2/3, rc_add1/1(ty)
  Delay1/1 -> Scope3/2, Subsystem/2(before_weight), Scope6/3
  Memory1/1 -> Weight/1, Scope5/2
  From Workspace7/1 -> rc_add1/2(initial_LTD)
  From Workspace9/1 -> rc_add1/3(tau_LTD)
  From Workspace6/1 -> rc_add2/2(initial_LTP)
  From Workspace8/1 -> rc_add2/3(tau_LTP)
  Product6/1 -> Scope1/4, Add1/2
  Product5/1 -> Scope1/2, Add1/1
  Add1/1 -> Subsystem/1(delta_weight), Scope2/1, Scope6/1
  From Workspace2/1 -> Product3/2
  Product2/1 -> Exp1/1
  Gain1/1 -> Product1/2, Product2/1
  From Workspace1/1 -> Switch1/3
  Exp1/1 -> Scope8/2, Product4/2
  Switch/1 -> Scope8/4, Switch1/2, Scope7/2, Switch1/1
  From Workspace3/1 -> Product2/2
  Product3/1 -> Switch/1
  Exp/1 -> Product3/1
  Clock3/1(T) -> Gain1/1
  Product1/1 -> Exp/1
  MATLAB Function1/1(y) -> Scope6/2, Product4/1, Scope7/1, Switch/2, Scope8/1
  From Workspace4/1 -> Product1/1
  From Workspace/1 -> MATLAB Function1/1(init_weight)
  Product4/1 -> Scope8/3, Switch/3
  Subsystem/1(weight) -> MATLAB Function1/3(before_weight)
  rc_add2/1(pre_trace) -> Product5/1, Scope1/1
  rc_add1/1(post_trace) -> Product6/2, Scope1/3
  OR/1 -> Subsystem/Trigger
  Memory2/1 -> OR/2, Product5/2, Clock2/1("Reset "), Scope2/5
  Pre_spike/1 -> OR/1, Scope5/1, Spike_out/1, Product/1, Clock3/1("Reset "), Clock1/1("Reset "), Product6/1, Scope2/2

== system stdp_pattern3x3_training_2023noclock/Synapse31 ==
  note: weight 초기값
  note: pre spike trace
  note: weight 최댓값
  note: STDP
  note: Synapse
  note: weight 최솟값
  note: post spike trace
  note: 기존 weight + STDP 변화량
  note: weight RC 감소
  Pre_spike : Inport
  addr : Inport  Port=2
  Post_spike : Inport  Port=3
  Add1 : Sum
  Clock1 : Subsystem
  Clock2 : Subsystem
  Clock3 : Subsystem
  Delay1 : Delay  DelayLength=1  SampleTime=0.00001
  Exp : Math
  Exp1 : Math
  From Workspace : FromWorkspace  VariableName=Rand_var
  From Workspace1 : FromWorkspace  VariableName=min_weight
  From Workspace2 : FromWorkspace  VariableName=max_weight
  From Workspace3 : FromWorkspace  VariableName=synapse_weight_rc_s
  From Workspace4 : FromWorkspace  VariableName=synapse_weight_rc_l
  From Workspace6 : FromWorkspace  VariableName=initial_LTP
  From Workspace7 : FromWorkspace  VariableName=initial_LTD
  From Workspace8 : FromWorkspace  VariableName=RC_LTP
  From Workspace9 : FromWorkspace  VariableName=RC_LTD
  Gain1 : Gain  Gain=-1
  MATLAB Function1 : MATLAB Function  TreatAsAtomicUnit=on
  Memory1 : Memory
  Memory2 : Memory
  OR : Logic  Operator=OR  IconShape=distinctive  AllPortsSameDT=off  OutDataTypeStr=boolean
  Product{,1..6} (7 alike) : Product
  Scope1 : Scope  NumInputPorts=4
  Scope2 : Scope  NumInputPorts=5
  Scope3 : Scope  NumInputPorts=2
  Scope5 : Scope  NumInputPorts=3
  Scope6 : Scope  NumInputPorts=3
  Scope7 : Scope  NumInputPorts=3
  Scope8 : Scope  NumInputPorts=4
  Subsystem : Subsystem
  Switch : Switch  Threshold=max_weight2  SaturateOnIntegerOverflow=off  InputSameDT=off
  Switch1 : Switch  Criteria=u2 > Threshold  Threshold=min_weight2  SaturateOnIntegerOverflow=off  InputSameDT=off
  rc_add1 : MATLAB Function  TreatAsAtomicUnit=on
  rc_add2 : MATLAB Function  TreatAsAtomicUnit=on
  Weight : Outport
  Spike_out : Outport  Port=2
  Weight_out : Outport  Port=3
  wires:
  Switch1/1 -> Scope7/3, Product/2, Weight_out/1, Scope5/3, Scope3/1, Delay1/1
  Product/1 -> Memory1/1
  addr/1 -> MATLAB Function1/2(synapse_num)
  Post_spike/1 -> Scope2/4, Memory2/1
  Clock1/1(T) -> rc_add2/1(tx)
  Clock2/1(T) -> Scope2/3, rc_add1/1(ty)
  Delay1/1 -> Scope3/2, Subsystem/2(before_weight), Scope6/3
  Memory1/1 -> Weight/1, Scope5/2
  From Workspace7/1 -> rc_add1/2(initial_LTD)
  From Workspace9/1 -> rc_add1/3(tau_LTD)
  From Workspace6/1 -> rc_add2/2(initial_LTP)
  From Workspace8/1 -> rc_add2/3(tau_LTP)
  Product6/1 -> Scope1/4, Add1/2
  Product5/1 -> Scope1/2, Add1/1
  Add1/1 -> Subsystem/1(delta_weight), Scope2/1, Scope6/1
  From Workspace2/1 -> Product3/2
  Product2/1 -> Exp1/1
  Gain1/1 -> Product1/2, Product2/1
  From Workspace1/1 -> Switch1/3
  Exp1/1 -> Scope8/2, Product4/2
  Switch/1 -> Scope8/4, Switch1/2, Scope7/2, Switch1/1
  From Workspace3/1 -> Product2/2
  Product3/1 -> Switch/1
  Exp/1 -> Product3/1
  Clock3/1(T) -> Gain1/1
  Product1/1 -> Exp/1
  MATLAB Function1/1(y) -> Scope6/2, Product4/1, Scope7/1, Switch/2, Scope8/1
  From Workspace4/1 -> Product1/1
  From Workspace/1 -> MATLAB Function1/1(init_weight)
  Product4/1 -> Scope8/3, Switch/3
  Subsystem/1(weight) -> MATLAB Function1/3(before_weight)
  rc_add2/1(pre_trace) -> Product5/1, Scope1/1
  rc_add1/1(post_trace) -> Product6/2, Scope1/3
  OR/1 -> Subsystem/Trigger
  Memory2/1 -> OR/2, Product5/2, Clock2/1("Reset "), Scope2/5
  Pre_spike/1 -> OR/1, Scope5/1, Spike_out/1, Product/1, Clock3/1("Reset "), Clock1/1("Reset "), Product6/1, Scope2/2

== system stdp_pattern3x3_training_2023noclock/Synapse32 ==
  note: weight 초기값
  note: pre spike trace
  note: weight 최댓값
  note: STDP
  note: Synapse
  note: weight 최솟값
  note: post spike trace
  note: 기존 weight + STDP 변화량
  note: weight RC 감소
  Pre_spike : Inport
  addr : Inport  Port=2
  Post_spike : Inport  Port=3
  Add1 : Sum
  Clock1 : Subsystem
  Clock2 : Subsystem
  Clock3 : Subsystem
  Delay1 : Delay  DelayLength=1  SampleTime=0.00001
  Exp : Math
  Exp1 : Math
  From Workspace : FromWorkspace  VariableName=Rand_var
  From Workspace1 : FromWorkspace  VariableName=min_weight
  From Workspace2 : FromWorkspace  VariableName=max_weight
  From Workspace3 : FromWorkspace  VariableName=synapse_weight_rc_s
  From Workspace4 : FromWorkspace  VariableName=synapse_weight_rc_l
  From Workspace6 : FromWorkspace  VariableName=initial_LTP
  From Workspace7 : FromWorkspace  VariableName=initial_LTD
  From Workspace8 : FromWorkspace  VariableName=RC_LTP
  From Workspace9 : FromWorkspace  VariableName=RC_LTD
  Gain1 : Gain  Gain=-1
  MATLAB Function1 : MATLAB Function  TreatAsAtomicUnit=on
  Memory1 : Memory
  Memory2 : Memory
  OR : Logic  Operator=OR  IconShape=distinctive  AllPortsSameDT=off  OutDataTypeStr=boolean
  Product{,1..6} (7 alike) : Product
  Scope1 : Scope  NumInputPorts=4
  Scope2 : Scope  NumInputPorts=5
  Scope3 : Scope  NumInputPorts=2
  Scope5 : Scope  NumInputPorts=3
  Scope6 : Scope  NumInputPorts=3
  Scope7 : Scope  NumInputPorts=3
  Scope8 : Scope  NumInputPorts=4
  Subsystem : Subsystem
  Switch : Switch  Threshold=max_weight2  SaturateOnIntegerOverflow=off  InputSameDT=off
  Switch1 : Switch  Criteria=u2 > Threshold  Threshold=min_weight2  SaturateOnIntegerOverflow=off  InputSameDT=off
  rc_add1 : MATLAB Function  TreatAsAtomicUnit=on
  rc_add2 : MATLAB Function  TreatAsAtomicUnit=on
  Weight : Outport
  Spike_out : Outport  Port=2
  Weight_out : Outport  Port=3
  wires:
  Switch1/1 -> Scope7/3, Product/2, Weight_out/1, Scope5/3, Scope3/1, Delay1/1
  Product/1 -> Memory1/1
  addr/1 -> MATLAB Function1/2(synapse_num)
  Post_spike/1 -> Scope2/4, Memory2/1
  Clock1/1(T) -> rc_add2/1(tx)
  Clock2/1(T) -> Scope2/3, rc_add1/1(ty)
  Delay1/1 -> Scope3/2, Subsystem/2(before_weight), Scope6/3
  Memory1/1 -> Weight/1, Scope5/2
  From Workspace7/1 -> rc_add1/2(initial_LTD)
  From Workspace9/1 -> rc_add1/3(tau_LTD)
  From Workspace6/1 -> rc_add2/2(initial_LTP)
  From Workspace8/1 -> rc_add2/3(tau_LTP)
  Product6/1 -> Scope1/4, Add1/2
  Product5/1 -> Scope1/2, Add1/1
  Add1/1 -> Subsystem/1(delta_weight), Scope2/1, Scope6/1
  From Workspace2/1 -> Product3/2
  Product2/1 -> Exp1/1
  Gain1/1 -> Product1/2, Product2/1
  From Workspace1/1 -> Switch1/3
  Exp1/1 -> Scope8/2, Product4/2
  Switch/1 -> Scope8/4, Switch1/2, Scope7/2, Switch1/1
  From Workspace3/1 -> Product2/2
  Product3/1 -> Switch/1
  Exp/1 -> Product3/1
  Clock3/1(T) -> Gain1/1
  Product1/1 -> Exp/1
  MATLAB Function1/1(y) -> Scope6/2, Product4/1, Scope7/1, Switch/2, Scope8/1
  From Workspace4/1 -> Product1/1
  From Workspace/1 -> MATLAB Function1/1(init_weight)
  Product4/1 -> Scope8/3, Switch/3
  Subsystem/1(weight) -> MATLAB Function1/3(before_weight)
  rc_add2/1(pre_trace) -> Product5/1, Scope1/1
  rc_add1/1(post_trace) -> Product6/2, Scope1/3
  OR/1 -> Subsystem/Trigger
  Memory2/1 -> OR/2, Product5/2, Clock2/1("Reset "), Scope2/5
  Pre_spike/1 -> OR/1, Scope5/1, Spike_out/1, Product/1, Clock3/1("Reset "), Clock1/1("Reset "), Product6/1, Scope2/2

== system stdp_pattern3x3_training_2023noclock/Synapse33 ==
  note: weight 초기값
  note: pre spike trace
  note: weight 최댓값
  note: STDP
  note: Synapse
  note: weight 최솟값
  note: post spike trace
  note: 기존 weight + STDP 변화량
  note: weight RC 감소
  Pre_spike : Inport
  addr : Inport  Port=2
  Post_spike : Inport  Port=3
  Add1 : Sum
  Clock1 : Subsystem
  Clock2 : Subsystem
  Clock3 : Subsystem
  Delay1 : Delay  DelayLength=1  SampleTime=0.00001
  Exp : Math
  Exp1 : Math
  From Workspace : FromWorkspace  VariableName=Rand_var
  From Workspace1 : FromWorkspace  VariableName=min_weight
  From Workspace2 : FromWorkspace  VariableName=max_weight
  From Workspace3 : FromWorkspace  VariableName=synapse_weight_rc_s
  From Workspace4 : FromWorkspace  VariableName=synapse_weight_rc_l
  From Workspace6 : FromWorkspace  VariableName=initial_LTP
  From Workspace7 : FromWorkspace  VariableName=initial_LTD
  From Workspace8 : FromWorkspace  VariableName=RC_LTP
  From Workspace9 : FromWorkspace  VariableName=RC_LTD
  Gain1 : Gain  Gain=-1
  MATLAB Function1 : MATLAB Function  TreatAsAtomicUnit=on
  Memory1 : Memory
  Memory2 : Memory
  OR : Logic  Operator=OR  IconShape=distinctive  AllPortsSameDT=off  OutDataTypeStr=boolean
  Product{,1..6} (7 alike) : Product
  Scope1 : Scope  NumInputPorts=4
  Scope2 : Scope  NumInputPorts=5
  Scope3 : Scope  NumInputPorts=2
  Scope5 : Scope  NumInputPorts=3
  Scope6 : Scope  NumInputPorts=3
  Scope7 : Scope  NumInputPorts=3
  Scope8 : Scope  NumInputPorts=4
  Subsystem : Subsystem
  Switch : Switch  Threshold=max_weight2  SaturateOnIntegerOverflow=off  InputSameDT=off
  Switch1 : Switch  Criteria=u2 > Threshold  Threshold=min_weight2  SaturateOnIntegerOverflow=off  InputSameDT=off
  rc_add1 : MATLAB Function  TreatAsAtomicUnit=on
  rc_add2 : MATLAB Function  TreatAsAtomicUnit=on
  Weight : Outport
  Spike_out : Outport  Port=2
  Weight_out : Outport  Port=3
  wires:
  Switch1/1 -> Scope7/3, Product/2, Weight_out/1, Scope5/3, Scope3/1, Delay1/1
  Product/1 -> Memory1/1
  addr/1 -> MATLAB Function1/2(synapse_num)
  Post_spike/1 -> Scope2/4, Memory2/1
  Clock1/1(T) -> rc_add2/1(tx)
  Clock2/1(T) -> Scope2/3, rc_add1/1(ty)
  Delay1/1 -> Scope3/2, Subsystem/2(before_weight), Scope6/3
  Memory1/1 -> Weight/1, Scope5/2
  From Workspace7/1 -> rc_add1/2(initial_LTD)
  From Workspace9/1 -> rc_add1/3(tau_LTD)
  From Workspace6/1 -> rc_add2/2(initial_LTP)
  From Workspace8/1 -> rc_add2/3(tau_LTP)
  Product6/1 -> Scope1/4, Add1/2
  Product5/1 -> Scope1/2, Add1/1
  Add1/1 -> Subsystem/1(delta_weight), Scope2/1, Scope6/1
  From Workspace2/1 -> Product3/2
  Product2/1 -> Exp1/1
  Gain1/1 -> Product1/2, Product2/1
  From Workspace1/1 -> Switch1/3
  Exp1/1 -> Scope8/2, Product4/2
  Switch/1 -> Scope8/4, Switch1/2, Scope7/2, Switch1/1
  From Workspace3/1 -> Product2/2
  Product3/1 -> Switch/1
  Exp/1 -> Product3/1
  Clock3/1(T) -> Gain1/1
  Product1/1 -> Exp/1
  MATLAB Function1/1(y) -> Scope6/2, Product4/1, Scope7/1, Switch/2, Scope8/1
  From Workspace4/1 -> Product1/1
  From Workspace/1 -> MATLAB Function1/1(init_weight)
  Product4/1 -> Scope8/3, Switch/3
  Subsystem/1(weight) -> MATLAB Function1/3(before_weight)
  rc_add2/1(pre_trace) -> Product5/1, Scope1/1
  rc_add1/1(post_trace) -> Product6/2, Scope1/3
  OR/1 -> Subsystem/Trigger
  Memory2/1 -> OR/2, Product5/2, Clock2/1("Reset "), Scope2/5
  Pre_spike/1 -> OR/1, Scope5/1, Spike_out/1, Product/1, Clock3/1("Reset "), Clock1/1("Reset "), Product6/1, Scope2/2

== system stdp_pattern3x3_training_2023noclock/Synapse34 ==
  note: weight 초기값
  note: pre spike trace
  note: weight 최댓값
  note: STDP
  note: Synapse
  note: weight 최솟값
  note: post spike trace
  note: 기존 weight + STDP 변화량
  note: weight RC 감소
  Pre_spike : Inport
  addr : Inport  Port=2
  Post_spike : Inport  Port=3
  Add1 : Sum
  Clock1 : Subsystem
  Clock2 : Subsystem
  Clock3 : Subsystem
  Delay1 : Delay  DelayLength=1  SampleTime=0.00001
  Exp : Math
  Exp1 : Math
  From Workspace : FromWorkspace  VariableName=Rand_var
  From Workspace1 : FromWorkspace  VariableName=min_weight
  From Workspace2 : FromWorkspace  VariableName=max_weight
  From Workspace3 : FromWorkspace  VariableName=synapse_weight_rc_s
  From Workspace4 : FromWorkspace  VariableName=synapse_weight_rc_l
  From Workspace6 : FromWorkspace  VariableName=initial_LTP
  From Workspace7 : FromWorkspace  VariableName=initial_LTD
  From Workspace8 : FromWorkspace  VariableName=RC_LTP
  From Workspace9 : FromWorkspace  VariableName=RC_LTD
  Gain1 : Gain  Gain=-1
  MATLAB Function1 : MATLAB Function  TreatAsAtomicUnit=on
  Memory1 : Memory
  Memory2 : Memory
  OR : Logic  Operator=OR  IconShape=distinctive  AllPortsSameDT=off  OutDataTypeStr=boolean
  Product{,1..6} (7 alike) : Product
  Scope1 : Scope  NumInputPorts=4
  Scope2 : Scope  NumInputPorts=5
  Scope3 : Scope  NumInputPorts=2
  Scope5 : Scope  NumInputPorts=3
  Scope6 : Scope  NumInputPorts=3
  Scope7 : Scope  NumInputPorts=3
  Scope8 : Scope  NumInputPorts=4
  Subsystem : Subsystem
  Switch : Switch  Threshold=max_weight2  SaturateOnIntegerOverflow=off  InputSameDT=off
  Switch1 : Switch  Criteria=u2 > Threshold  Threshold=min_weight2  SaturateOnIntegerOverflow=off  InputSameDT=off
  rc_add1 : MATLAB Function  TreatAsAtomicUnit=on
  rc_add2 : MATLAB Function  TreatAsAtomicUnit=on
  Weight : Outport
  Spike_out : Outport  Port=2
  Weight_out : Outport  Port=3
  wires:
  Switch1/1 -> Scope7/3, Product/2, Weight_out/1, Scope5/3, Scope3/1, Delay1/1
  Product/1 -> Memory1/1
  addr/1 -> MATLAB Function1/2(synapse_num)
  Post_spike/1 -> Scope2/4, Memory2/1
  Clock1/1(T) -> rc_add2/1(tx)
  Clock2/1(T) -> Scope2/3, rc_add1/1(ty)
  Delay1/1 -> Scope3/2, Subsystem/2(before_weight), Scope6/3
  Memory1/1 -> Weight/1, Scope5/2
  From Workspace7/1 -> rc_add1/2(initial_LTD)
  From Workspace9/1 -> rc_add1/3(tau_LTD)
  From Workspace6/1 -> rc_add2/2(initial_LTP)
  From Workspace8/1 -> rc_add2/3(tau_LTP)
  Product6/1 -> Scope1/4, Add1/2
  Product5/1 -> Scope1/2, Add1/1
  Add1/1 -> Subsystem/1(delta_weight), Scope2/1, Scope6/1
  From Workspace2/1 -> Product3/2
  Product2/1 -> Exp1/1
  Gain1/1 -> Product1/2, Product2/1
  From Workspace1/1 -> Switch1/3
  Exp1/1 -> Scope8/2, Product4/2
  Switch/1 -> Scope8/4, Switch1/2, Scope7/2, Switch1/1
  From Workspace3/1 -> Product2/2
  Product3/1 -> Switch/1
  Exp/1 -> Product3/1
  Clock3/1(T) -> Gain1/1
  Product1/1 -> Exp/1
  MATLAB Function1/1(y) -> Scope6/2, Product4/1, Scope7/1, Switch/2, Scope8/1
  From Workspace4/1 -> Product1/1
  From Workspace/1 -> MATLAB Function1/1(init_weight)
  Product4/1 -> Scope8/3, Switch/3
  Subsystem/1(weight) -> MATLAB Function1/3(before_weight)
  rc_add2/1(pre_trace) -> Product5/1, Scope1/1
  rc_add1/1(post_trace) -> Product6/2, Scope1/3
  OR/1 -> Subsystem/Trigger
  Memory2/1 -> OR/2, Product5/2, Clock2/1("Reset "), Scope2/5
  Pre_spike/1 -> OR/1, Scope5/1, Spike_out/1, Product/1, Clock3/1("Reset "), Clock1/1("Reset "), Product6/1, Scope2/2
